simulink model "TaktgesteuerterZaehler4bit"  (R2018a)
settings: Solver=VariableStepAuto  StartTime=0.0  StopTime=10.0  RelTol=1e-3
libraries: simulink_extras x5
settings Model: Creator=SV-97  LastModifiedBy=SV-97

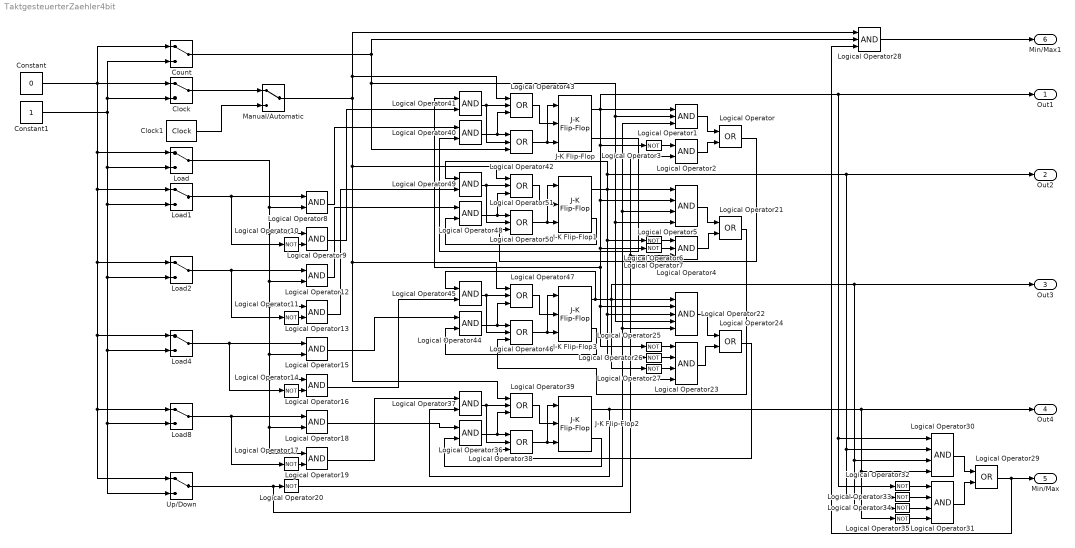
== system TaktgesteuerterZaehler4bit ==
  Clock : ManualSwitch
  Clock1 : simulink_extras/Flip Flops/Clock  period=5
  Constant : Constant  Value=0
  Constant1 : Constant
  Count : ManualSwitch
  J-K Flip-Flop{,1..3} (4 alike) : simulink_extras/Flip Flops/J-K Flip-Flop  initial_condition=0
      settings: SourceProductName=Simulink
  Load{,1..2,4,8} (5 alike) : ManualSwitch
  Logical Operator{,21,24,29} (4 alike) : Logic  Operator=OR  AllPortsSameDT=off  OutDataTypeStr=boolean
  Logical Operator1 : Logic  Inputs=3  AllPortsSameDT=off  OutDataTypeStr=boolean
  Logical Operator{3,6..7,10..11,14,17,20,25..27,32..35} (15 alike) : Logic  Operator=NOT  AllPortsSameDT=off  OutDataTypeStr=boolean
  Logical Operator{2,8..9,12..13,15..16,18..19,36..37,40..41,44..45,48..49} (17 alike) : Logic  AllPortsSameDT=off  OutDataTypeStr=boolean
  Logical Operator22 : Logic  Inputs=5  AllPortsSameDT=off  OutDataTypeStr=boolean
  Logical Operator{5,23,30..31} (4 alike) : Logic  Inputs=4  AllPortsSameDT=off  OutDataTypeStr=boolean
  Logical Operator28 : Logic  Inputs=3  AllPortsSameDT=off  OutDataTypeStr=boolean
  Logical Operator{38..39,42..43,46..47,50..51} (8 alike) : Logic  Operator=OR  Inputs=3  AllPortsSameDT=off  OutDataTypeStr=boolean
  Logical Operator4 : Logic  Inputs=3  AllPortsSameDT=off  OutDataTypeStr=boolean
  Manual/Automatic : ManualSwitch
  Up/Down : ManualSwitch
  Out1 : Outport
  Out2 : Outport  Port=2
  Out3 : Outport  Port=3
  Out4 : Outport  Port=4
  Min/Max : Outport  Port=5
  Min/Max1 : Outport  Port=6
  wires:
  Count/1 -> Logical Operator22/4, Logical Operator5/4, Logical Operator1/2, Logical Operator42/3, Logical Operator28/2
  Manual/Automatic/1 -> Logical Operator51/1, Logical Operator47/1, Logical Operator39/1, Logical Operator43/1, Logical Operator28/1
  Logical Operator1/1 -> Logical Operator/1
  Logical Operator2/1 -> Logical Operator/2
  Logical Operator3/1 -> Logical Operator2/1
  J-K Flip-Flop/1 -> Logical Operator41/1, Logical Operator25/1, Logical Operator22/2, Logical Operator7/1, Logical Operator5/2, Logical Operator3/1, Out1/1, Logical Operator30/1, Logical Operator32/1, Logical Operator1/1
  Logical Operator6/1 -> Logical Operator4/1
  Logical Operator7/1 -> Logical Operator4/2
  J-K Flip-Flop1/1 -> Logical Operator49/1, Logical Operator33/1, Logical Operator30/2, Out2/1, Logical Operator5/1, Logical Operator26/1, Logical Operator22/3, Logical Operator6/1
  Logical Operator10/1 -> Logical Operator9/2
  Logical Operator11/1 -> Logical Operator13/2
  Logical Operator14/1 -> Logical Operator16/2
  Logical Operator17/1 -> Logical Operator19/2
  Load/1 -> Logical Operator19/1, Logical Operator18/2, Logical Operator16/1, Logical Operator15/2, Logical Operator13/1, Logical Operator12/2, Logical Operator9/1, Logical Operator8/2
  Load1/1 -> Logical Operator10/1, Logical Operator8/1
  Load2/1 -> Logical Operator11/1, Logical Operator12/1
  Load4/1 -> Logical Operator14/1, Logical Operator15/1
  Load8/1 -> Logical Operator17/1, Logical Operator18/1
  Up/Down/1 -> Logical Operator2/2, Logical Operator4/3, Logical Operator23/4, Logical Operator20/1
  Logical Operator5/1 -> Logical Operator21/1
  Logical Operator4/1 -> Logical Operator21/2
  Logical Operator20/1 -> Logical Operator1/3, Logical Operator5/3, Logical Operator22/5
  Logical Operator22/1 -> Logical Operator24/1
  Logical Operator23/1 -> Logical Operator24/2
  J-K Flip-Flop3/1 -> Logical Operator45/1, Logical Operator27/1, Out3/1, Logical Operator34/1, Logical Operator30/3, Logical Operator22/1
  Logical Operator25/1 -> Logical Operator23/1
  Logical Operator26/1 -> Logical Operator23/2
  Logical Operator27/1 -> Logical Operator23/3
  J-K Flip-Flop2/1 -> Logical Operator37/2, Logical Operator35/1, Logical Operator30/4, Out4/1
  Logical Operator34/1 -> Logical Operator31/3
  Logical Operator32/1 -> Logical Operator31/1
  Logical Operator33/1 -> Logical Operator31/2
  Logical Operator35/1 -> Logical Operator31/4
  Logical Operator31/1 -> Logical Operator29/2
  Logical Operator30/1 -> Logical Operator29/1
  Logical Operator29/1 -> Logical Operator28/3, Min/Max/1
  Logical Operator28/1 -> Min/Max1/1
  Logical Operator36/1 -> Logical Operator39/3, Logical Operator38/1
  Logical Operator39/1 -> J-K Flip-Flop2/2
  Logical Operator38/1 -> J-K Flip-Flop2/1, J-K Flip-Flop2/3
  J-K Flip-Flop2/2 -> Logical Operator36/2
  Logical Operator24/1 -> Logical Operator38/3
  Logical Operator18/1 -> Logical Operator36/1
  Logical Operator37/1 -> Logical Operator38/2, Logical Operator39/2
  Logical Operator19/1 -> Logical Operator37/1
  Logical Operator43/1 -> J-K Flip-Flop/2
  Logical Operator41/1 -> Logical Operator42/2, Logical Operator43/2
  Logical Operator42/1 -> J-K Flip-Flop/1, J-K Flip-Flop/3
  Logical Operator40/1 -> Logical Operator43/3, Logical Operator42/1
  Logical Operator46/1 -> J-K Flip-Flop3/1, J-K Flip-Flop3/3
  Logical Operator44/1 -> Logical Operator47/3, Logical Operator46/1
  Logical Operator45/1 -> Logical Operator46/2, Logical Operator47/2
  Logical Operator47/1 -> J-K Flip-Flop3/2
  Logical Operator50/1 -> J-K Flip-Flop1/3, J-K Flip-Flop1/1
  Logical Operator48/1 -> Logical Operator51/3, Logical Operator50/1
  Logical Operator49/1 -> Logical Operator50/2, Logical Operator51/2
  Logical Operator51/1 -> J-K Flip-Flop1/2
  J-K Flip-Flop3/2 -> Logical Operator44/2
  Logical Operator21/1 -> Logical Operator46/3
  Logical Operator16/1 -> Logical Operator45/2
  Logical Operator15/1 -> Logical Operator44/1
  Logical Operator/1 -> Logical Operator50/3
  Logical Operator13/1 -> Logical Operator49/2
  Logical Operator12/1 -> Logical Operator48/1
  J-K Flip-Flop1/2 -> Logical Operator48/2
  J-K Flip-Flop/2 -> Logical Operator40/2
  Logical Operator9/1 -> Logical Operator41/2
  Logical Operator8/1 -> Logical Operator40/1
  Constant/1 -> Clock/1, Up/Down/1, Load8/1, Load4/1, Load2/1, Load1/1, Load/1, Count/1
  Constant1/1 -> Up/Down/2, Load8/2, Load4/2, Load2/2, Load1/2, Load/2, Clock/2, Count/2
  Clock/1 -> Manual/Automatic/1
  Clock1/1 -> Manual/Automatic/2
